simulink model "combined_system"  (R2023a)
settings: Solver=VariableStepAuto  StartTime=0.0  StopTime=6  RelTol=1e-3
libraries: simulink x4
settings Model: Creator=Gizem  LastModifiedBy=Gizem
settings SolverCC: ZeroCrossAlgorithm=Adaptive
settings DebuggingCC: IgnoredZcDiagnostic=none

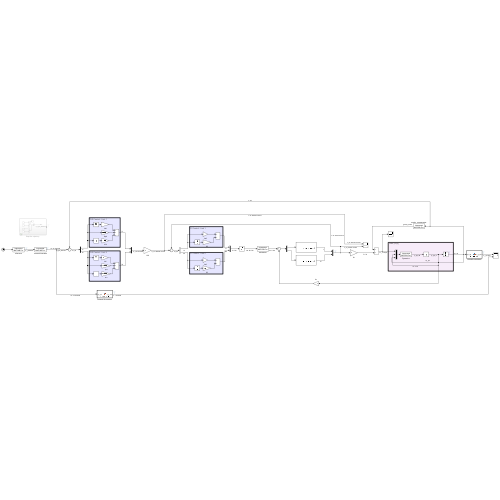
[thumbnail: Simulink's stored preview of the top-level diagram]
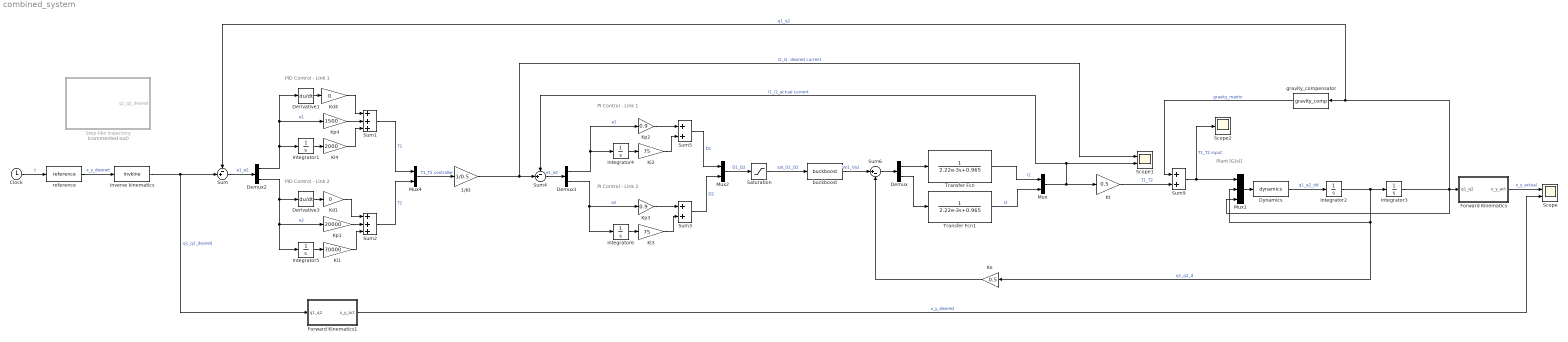
== system combined_system ==
  note: PID Control - Link 2
  note: PID Control - Link 1
  note: Plant [G(s)]
  note: PI Control - Link 2
  note: PI Control - Link 1
  1/Kt : Gain  Gain=1/0.5
  Clock : Clock
  Demux : Demux  Outputs=2
  Demux1 : Demux  Outputs=2
  Demux2 : Demux  Outputs=2
  Derivative1 : Derivative
  Derivative3 : Derivative
  Dynamics : MATLABFcn  MATLABFcn=dynamics  OutputDimensions=2
  Forward Kinematics : MATLAB Function  TreatAsAtomicUnit=on
  Forward Kinematics1 : MATLAB Function  TreatAsAtomicUnit=on
  Integrator{1,4..6} (4 alike) : Integrator
  Integrator2 : Integrator  InitialCondition=[0 0]
  Integrator3 : Integrator  InitialCondition=[0 0]
  Kd1 : Gain  Gain=0
  Kd4 : Gain  Gain=0
  Ke : Gain  Gain=0.5
  Ki1 : Gain  Gain=70000
  Ki2 : Gain  Gain=75
  Ki3 : Gain  Gain=75
  Ki4 : Gain  Gain=2000
  Kp1 : Gain  Gain=20000
  Kp2 : Gain  Gain=0.9
  Kp3 : Gain  Gain=0.9
  Kp4 : Gain  Gain=1500
  Kt : Gain  Gain=0.5
  Mux : Mux  Inputs=2
  Mux1 : Mux  Inputs=3
  Mux2 : Mux  Inputs=2
  Mux4 : Mux  Inputs=2
  Saturation : Saturate  UpperLimit=0.8  LowerLimit=-0.8
  Scope : Scope  NumInputPorts=2
  Scope1 : Scope  NumInputPorts=2
  Scope2 : Scope
  Step-like trajectory : Subsystem  Commented=on
  Sum : Sum  Inputs=-+|
  Sum1 : Sum  Inputs=+++
  Sum2 : Sum  Inputs=+++
  Sum3 : Sum
  Sum4 : Sum  Inputs=-+|
  Sum5 : Sum
  Sum6 : Sum  Inputs=|+-
  Sum9 : Sum
  Transfer Fcn : TransferFcn  Denominator=[2.22e-3 0.965]
  Transfer Fcn1 : TransferFcn  Denominator=[2.22e-3 0.965]
  buckboost : MATLABFcn  MATLABFcn=buckboost  OutputDimensions=2
  gravity_compensator : MATLABFcn  MATLABFcn=gravity_comp  OutputDimensions=2
  inverse kinematics : MATLABFcn  MATLABFcn=invkine  OutputDimensions=2
  reference : MATLABFcn  MATLABFcn=reference  OutputDimensions=2
  wires:
  inverse kinematics/1 -> Sum/2, Forward Kinematics1/1(q1_q2)  "q1_q2_desired"
  reference/1 -> inverse kinematics/1  "x_y_desired"
  Demux2/1 -> Kp4/1, Derivative1/1, Integrator1/1  "e1"
  Clock/1 -> reference/1  "t"
  Sum1/1 -> Mux4/1  "T1"
  Integrator2/1 -> Mux1/2, Ke/1, Integrator3/1  "q1_q2_d"
  Ki1/1 -> Sum2/3
  Kd1/1 -> Sum2/1
  Dynamics/1 -> Integrator2/1  "q1_q2_dd"
  Sum2/1 -> Mux4/2  "T2"
  Derivative1/1 -> Kd4/1
  Forward Kinematics1/1(x_y_act) -> Scope/2  "x_y_desired"
  Demux2/2 -> Kp1/1, Integrator5/1, Derivative3/1  "e2"
  Kp1/1 -> Sum2/2
  Integrator5/1 -> Ki1/1
  Kd4/1 -> Sum1/1
  Ki4/1 -> Sum1/3
  Integrator1/1 -> Ki4/1
  Integrator3/1 -> Mux1/3, Forward Kinematics/1(q1_q2), gravity_compensator/1, Sum/1  "q1_q2"
  Kp4/1 -> Sum1/2
  Mux1/1 -> Dynamics/1
  Sum9/1 -> Scope2/1, Mux1/1  "T1_T2 input"
  Mux4/1 -> 1/Kt/1  "T1_T2 controller"
  Forward Kinematics/1(x_y_act) -> Scope/1  "x_y_actual"
  Sum/1 -> Demux2/1  "e1_e2"
  Derivative3/1 -> Kd1/1
  gravity_compensator/1 -> Sum9/1  "gravity_matrix"
  Integrator6/1 -> Ki3/1
  Ki3/1 -> Sum3/2
  Sum5/1 -> Mux2/1  "D1"
  Integrator4/1 -> Ki2/1
  Sum3/1 -> Mux2/2  "D2"
  Demux/1 -> Transfer Fcn/1
  Demux/2 -> Transfer Fcn1/1
  Mux2/1 -> Saturation/1  "D1_D2"
  Sum6/1 -> Demux/1
  Kp3/1 -> Sum3/1
  Sum4/1 -> Demux1/1  "e1_e2"
  buckboost/1 -> Sum6/1  "Vo1_Vo2"
  Demux1/2 -> Integrator6/1, Kp3/1  "e2"
  Kp2/1 -> Sum5/1
  Ki2/1 -> Sum5/2
  Saturation/1 -> buckboost/1  "sat_D1_D2"
  Demux1/1 -> Integrator4/1, Kp2/1  "e1"
  Transfer Fcn1/1 -> Mux/2  "I2"
  Mux/1 -> Kt/1, Sum4/1, Scope1/2  "I1_I2_actual current"
  1/Kt/1 -> Scope1/1, Sum4/2  "I1_I2  desired current"
  Transfer Fcn/1 -> Mux/1  "I1"
  Ke/1 -> Sum6/2
  Kt/1 -> Sum9/2  "T1_T2"

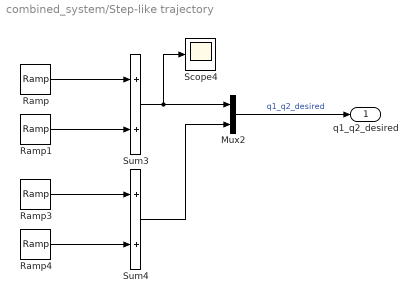
== system combined_system/Step-like trajectory ==
  Mux2 : Mux  Inputs=2
  Ramp : simulink/Sources/Ramp  slope=400  start=0  InitialOutput=0
  Ramp1 : simulink/Sources/Ramp  slope=-400  start=0.1  InitialOutput=0
  Ramp3 : simulink/Sources/Ramp  slope=400  start=0  InitialOutput=0
  Ramp4 : simulink/Sources/Ramp  slope=-400  start=0.1  InitialOutput=0
  Scope4 : Scope
  Sum3 : Sum
  Sum4 : Sum
  q1_q2_desired : Outport
  wires:
  Sum3/1 -> Scope4/1, Mux2/1
  Ramp1/1 -> Sum3/2
  Ramp3/1 -> Sum4/1
  Ramp4/1 -> Sum4/2
  Ramp/1 -> Sum3/1
  Sum4/1 -> Mux2/2
  Mux2/1 -> q1_q2_desired/1  "q1_q2_desired"

== matlab function combined_system/Forward Kinematics ==
  data: q1_q2 input; x_y_act output
function x_y_act = forwardkine(q1_q2)

    % shaft to shaft length of the links
    % link length 1 = 600mm = 0.6 m
    % link length 2 = 400mm = 0.4 m
    
    l1 = 0.6;
    l2 = 0.4;
    
    q1 = q1_q2(1);
    q2 = q1_q2(2);
    
    x1 = l1*cosd(q1);
    y1 = l1*sind(q1);
    
    x2 = x1 + l2*cosd(q1+q2);
    y2 = y1 + l2*sind(q1+q2);
    x_act = x2;
    y_act = y2;
    
    x_y_act = [x_act; y_act];
end

== matlab function combined_system/Forward Kinematics1 ==
  data: q1_q2 input; x_y_act output
function x_y_act = forwardkine(q1_q2)

% shaft to shaft length of the links
% link length 1 = 600mm = 0.6 m
% link length 2 = 400mm = 0.4 m

l1 = 0.6;
l2 = 0.4;

q1 = q1_q2(1);
q2 = q1_q2(2);

x1 = l1*cosd(q1);
y1 = l1*sind(q1);

x2 = x1 + l2*cosd(q1+q2);
y2 = y1 + l2*sind(q1+q2);
x_act = x2;
y_act = y2;

x_y_act = [x_act; y_act];
end
